simulink model "full_maneuver_platoon_new_strategy"  (R2019a)
settings: Solver=VariableStepAuto  StartTime=0.0  StopTime=70  FixedStep=0.1  MaxStep=0.05  RelTol=1e-3
libraries: simulink x97, dspsigops x7, powerlib_meascontrol x7, autolibshared x7
(part 1 of 7)
settings Model: Creator=fvall  LastModifiedBy=fvall

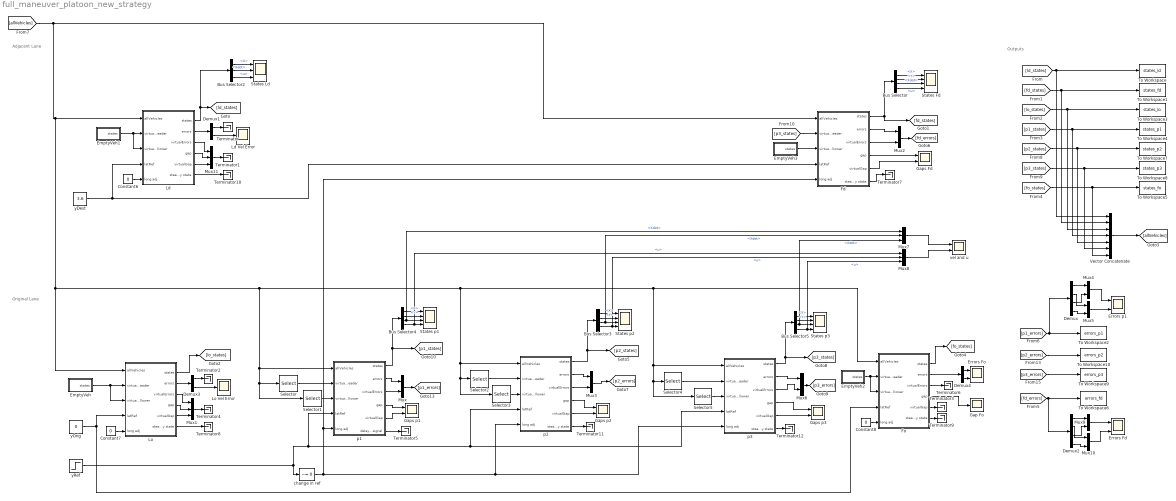
== system full_maneuver_platoon_new_strategy ==
  note: Adjacent Lane
  note: Outputs
  note: Original Lane
  Bus Selector{,3..5} (4 alike) : BusSelector  OutputSignals=X,Y,Xdot,u
  Bus Selector2 : BusSelector  OutputSignals=X,Xdot,u
  Constant6 : Constant  Value=0
  Constant7 : Constant  Value=0
  Constant8 : Constant  Value=0
  Demux : Demux
  Demux1 : Demux  Outputs=2
  Demux2 : Demux
  Demux3 : Demux  Outputs=2
  Demux4 : Demux  Outputs=2
  EmptyVeh : Subsystem
  EmptyVeh1 : Subsystem
  EmptyVeh2 : Subsystem
  EmptyVeh3 : Subsystem
  Errors Fd : Scope  NumInputPorts=2
  Errors Fo : Scope  NumInputPorts=2
  Errors p1 : Scope  NumInputPorts=2
  Fd : Subsystem  mask{m=2000, lf=2.5, lr=2.5, maxAcceleration=4, minAcceleration=-8, maxJerk=40, minJerk=-50, maxDelta=0.43633, maxDeltaDot=0.16406, freeFlowVel=29, A=[0 1 25 0;0 -0.92 0 -25.1;0 0 0 1;0 -0.05 0 -2.875], B=[0;12;0;15], C=[1 0 0 0;0 0 0 1], x0=40.2312, vx0=29, y0=3.6, h=0.63, d0=0.5004, minHeadwayError=-100, maxHeadwayError=3, velFilterGain=10, Kd=1.5652, Kp=2.2775, Ki=0.75, velKi=0.5, velKp=1.5, hFilterGain=0.5, vMin=18, maxComfAccel=2, minComfAccel=-2, maxComfJerk=10, minComfJerk=-10, hLc=2.1525, d0Lc=0.5004, Klat=[0.00909090909090922 0.00739381562390402 0.848484848484842 0.174418280834209], L=[12.1618468638973 6.0911647386398;-3.34743889176456 -72.8238882817198;1.29674659792577 4.97919690407453;0.0997536738638272 3.54315313610273]}
      mask prompts: m "autoblks_shared:autoblkVehBody3DofLat:blkPrm_m"; lf "autoblks_shared:autoblkVehBody3DofLat:blkPrm_a"; lr "autoblks_shared:autoblkVehBody3DofLat:blkPrm_b"; maxAcceleration "Max Acceleration"; minAcceleration "Min Acceleration"; maxJerk "Max Jerk"; minJerk "Min Jerk"; maxDelta "Max Delta"; maxDeltaDot "Max Delta Dot"; freeFlowVel "Free Flow Velocity"; x0 "autoblks_shared:autoblkVehBody3DofLat:blkPrm_X_o"; vx0 "autoblks_shared:autoblkVehBody3DofLat:blkPrm_xdot_o"; y0 "autoblks_shared:autoblkVehBody3DofLat:blkPrm_Y_o"; h "Time Headway"; d0 "Standstill Gap"; minHeadwayError "Min Headway Error"; maxHeadwayError "Max Headway Error"; velFilterGain "Velocity Filter Gain"; hFilterGain "Headway filter Gain"; vMin "Min velocity"; maxComfAccel "Max Comf Accel"; minComfAccel "Min Comf Accel"; maxComfJerk "Max Comf Jerk"; minComfJerk "Min Comf Jerk"; hLc "Time Headway LC"; d0Lc "Standstill Gap LC"; Klat "Lat Controller Gain"; L "Observer Gain"
      mask TypeOptions m: Vehicle Body 3DOF Single Track/m
      mask TypeOptions lf: Vehicle Body 3DOF Single Track/a
      mask TypeOptions lr: Vehicle Body 3DOF Single Track/b
      mask TypeOptions maxDelta: Lateral Control/Saturation/UpperLimit
      mask TypeOptions maxDeltaDot: Lateral Control/Rate Limiter/RisingSlewLimit
      mask TypeOptions A:
      | Lateral Control/Full State
      | Observer/Gain3/Gain
      mask TypeOptions B:
      | Lateral Control/Full State
      | Observer/Gain/Gain
      mask TypeOptions C:
      | Lateral Control/Full State
      | Observer/Gain1/Gain
      mask TypeOptions x0: Vehicle Body 3DOF Single Track/X_o
      mask TypeOptions vx0: Vehicle Body 3DOF Single Track/xdot_o
      mask TypeOptions y0: Vehicle Body 3DOF Single Track/Y_o
      mask TypeOptions h:
      | Regular Vehicle
      | Following/Compute Errors/h/Value
      mask TypeOptions d0:
      | Regular Vehicle
      | Following/Compute Errors/d0/Value
      mask TypeOptions Klat: Lateral Control/Gain1/Gain
      mask TypeOptions L:
      | Lateral Control/Full State
      | Observer/Gain2/Gain
      mask DialogControl DescGroupVar Prompt: 3DOF Vehicle with ACC
      mask DialogControl DescTextVar Prompt: Vehicle with ACC. The vehicle model is Simulink's 3DOF single track vehicle body. The controller is a PID with constant headway including headway error saturation and filtered leader velocity.
      mask DialogControl VehParams Prompt: Vehicle Parameters
      mask DialogControl m Prompt: Vehicle mass, m [kg]:
      mask DialogControl lf Prompt: Longitudinal distance from center of mass to front axle, a [m]:
      mask DialogControl lr Prompt: Longitudinal distance from center of mass to rear axle, b [m]:
      mask DialogControl latLinearModel Prompt: Lat Linear Model
      mask DialogControl InitStates Prompt: Initial State
      mask DialogControl x0 Prompt: Initial inertial frame longitudinal position, X_o [m]:
      mask DialogControl vx0 Prompt: Initial longitudinal velocity, xdot_o [m/s]:
      mask DialogControl y0 Prompt: Initial inertial frame lateral displacement, Y_o [m]:
      mask DialogControl Container3 Prompt: Veh Following Parameters
      mask DialogControl VirtualFollParams Prompt: Virtual Veh Following Parameters
      mask DialogControl LCParams Prompt: Lane Change Params
  Fo : Subsystem  mask{m=2000, lf=2.5, lr=2.5, maxAcceleration=4, minAcceleration=-8, maxJerk=40, minJerk=-50, maxDelta=0.43633, maxDeltaDot=0.16406, freeFlowVel=25, A=[0 1 25 0;0 -0.92 0 -25.1;0 0 0 1;0 -0.05 0 -2.875], B=[0;12;0;15], C=[1 0 0 0;0 0 0 1], x0=0, vx0=25, y0=0, h=0.63, d0=0.5004, minHeadwayError=-100, maxHeadwayError=3, velFilterGain=10, Kd=1.5652, Kp=2.2775, Ki=0.75, velKi=0.5, velKp=1.5, hFilterGain=0.5, vMin=18, maxComfAccel=2, minComfAccel=-2, maxComfJerk=10, minComfJerk=-10, hLc=1.9025, d0Lc=0.5004, Klat=[0.00909090909090922 0.00739381562390402 0.848484848484842 0.174418280834209], L=[12.1618468638973 6.0911647386398;-3.34743889176456 -72.8238882817198;1.29674659792577 4.97919690407453;0.0997536738638272 3.54315313610273]}
      mask prompts: m "autoblks_shared:autoblkVehBody3DofLat:blkPrm_m"; lf "autoblks_shared:autoblkVehBody3DofLat:blkPrm_a"; lr "autoblks_shared:autoblkVehBody3DofLat:blkPrm_b"; maxAcceleration "Max Acceleration"; minAcceleration "Min Acceleration"; maxJerk "Max Jerk"; minJerk "Min Jerk"; maxDelta "Max Delta"; maxDeltaDot "Max Delta Dot"; freeFlowVel "Free Flow Velocity"; x0 "autoblks_shared:autoblkVehBody3DofLat:blkPrm_X_o"; vx0 "autoblks_shared:autoblkVehBody3DofLat:blkPrm_xdot_o"; y0 "autoblks_shared:autoblkVehBody3DofLat:blkPrm_Y_o"; h "Time Headway"; d0 "Standstill Gap"; minHeadwayError "Min Headway Error"; maxHeadwayError "Max Headway Error"; velFilterGain "Velocity Filter Gain"; hFilterGain "Headway filter Gain"; vMin "Min velocity"; maxComfAccel "Max Comf Accel"; minComfAccel "Min Comf Accel"; maxComfJerk "Max Comf Jerk"; minComfJerk "Min Comf Jerk"; hLc "Time Headway LC"; d0Lc "Standstill Gap LC"; Klat "Lat Controller Gain"; L "Observer Gain"
      mask TypeOptions m: Vehicle Body 3DOF Single Track/m
      mask TypeOptions lf: Vehicle Body 3DOF Single Track/a
      mask TypeOptions lr: Vehicle Body 3DOF Single Track/b
      mask TypeOptions maxDelta: Lateral Control/Saturation/UpperLimit
      mask TypeOptions maxDeltaDot: Lateral Control/Rate Limiter/RisingSlewLimit
      mask TypeOptions A:
      | Lateral Control/Full State
      | Observer/Gain3/Gain
      mask TypeOptions B:
      | Lateral Control/Full State
      | Observer/Gain/Gain
      mask TypeOptions C:
      | Lateral Control/Full State
      | Observer/Gain1/Gain
      mask TypeOptions x0: Vehicle Body 3DOF Single Track/X_o
      mask TypeOptions vx0: Vehicle Body 3DOF Single Track/xdot_o
      mask TypeOptions y0: Vehicle Body 3DOF Single Track/Y_o
      mask TypeOptions h:
      | Regular Vehicle
      | Following/Compute Errors/h/Value
      mask TypeOptions d0:
      | Regular Vehicle
      | Following/Compute Errors/d0/Value
      mask TypeOptions vMin:
      | Longitudinal Adjustments
      | for Lane Change/Virtual Leader Following/vMin/Value
      mask TypeOptions Klat: Lateral Control/Gain1/Gain
      mask TypeOptions L:
      | Lateral Control/Full State
      | Observer/Gain2/Gain
      mask DialogControl DescGroupVar Prompt: 3DOF Vehicle with ACC
      mask DialogControl DescTextVar Prompt: Vehicle with ACC. The vehicle model is Simulink's 3DOF single track vehicle body. The controller is a PID with constant headway including headway error saturation and filtered leader velocity.
      mask DialogControl VehParams Prompt: Vehicle Parameters
      mask DialogControl m Prompt: Vehicle mass, m [kg]:
      mask DialogControl lf Prompt: Longitudinal distance from center of mass to front axle, a [m]:
      mask DialogControl lr Prompt: Longitudinal distance from center of mass to rear axle, b [m]:
      mask DialogControl latLinearModel Prompt: Lat Linear Model
      mask DialogControl InitStates Prompt: Initial State
      mask DialogControl x0 Prompt: Initial inertial frame longitudinal position, X_o [m]:
      mask DialogControl vx0 Prompt: Initial longitudinal velocity, xdot_o [m/s]:
      mask DialogControl y0 Prompt: Initial inertial frame lateral displacement, Y_o [m]:
      mask DialogControl Container3 Prompt: Veh Following Parameters
      mask DialogControl VirtualFollParams Prompt: Virtual Veh Following Parameters
      mask DialogControl LCParams Prompt: Lane Change Params
  Gap Fo : Scope
  Gaps Fd : Scope  NumInputPorts=2
  Gaps p1 : Scope  NumInputPorts=2
  Gaps p2 : Scope  NumInputPorts=2
  Gaps p3 : Scope  NumInputPorts=2
  Ld : Subsystem  mask{m=2000, lf=2.5, lr=2.5, maxAcceleration=4, minAcceleration=-8, maxJerk=40, minJerk=-50, maxDelta=0.43633, maxDeltaDot=0.16406, freeFlowVel=29, A=[0 1 25 0;0 -0.92 0 -25.1;0 0 0 1;0 -0.05 0 -2.875], B=[0;12;0;15], C=[1 0 0 0;0 0 0 1], x0=64.0016, vx0=29, y0=3.6, h=0.63, d0=0.5004, minHeadwayError=-100, maxHeadwayError=3, velFilterGain=10, Kd=1.5652, Kp=2.2775, Ki=0.75, velKi=0.5, velKp=1.5, hFilterGain=0.5, vMin=18, maxComfAccel=2, minComfAccel=-2, maxComfJerk=10, minComfJerk=-10, hLc=2.1525, d0Lc=0.5004, Klat=[0.00909090909090922 0.00739381562390402 0.848484848484842 0.174418280834209], L=[12.1618468638973 6.0911647386398;-3.34743889176456 -72.8238882817198;1.29674659792577 4.97919690407453;0.0997536738638272 3.54315313610273]}
      mask prompts: m "autoblks_shared:autoblkVehBody3DofLat:blkPrm_m"; lf "autoblks_shared:autoblkVehBody3DofLat:blkPrm_a"; lr "autoblks_shared:autoblkVehBody3DofLat:blkPrm_b"; maxAcceleration "Max Acceleration"; minAcceleration "Min Acceleration"; maxJerk "Max Jerk"; minJerk "Min Jerk"; maxDelta "Max Delta"; maxDeltaDot "Max Delta Dot"; freeFlowVel "Free Flow Velocity"; x0 "autoblks_shared:autoblkVehBody3DofLat:blkPrm_X_o"; vx0 "autoblks_shared:autoblkVehBody3DofLat:blkPrm_xdot_o"; y0 "autoblks_shared:autoblkVehBody3DofLat:blkPrm_Y_o"; h "Time Headway"; d0 "Standstill Gap"; minHeadwayError "Min Headway Error"; maxHeadwayError "Max Headway Error"; velFilterGain "Velocity Filter Gain"; hFilterGain "Headway filter Gain"; vMin "Min velocity"; maxComfAccel "Max Comf Accel"; minComfAccel "Min Comf Accel"; maxComfJerk "Max Comf Jerk"; minComfJerk "Min Comf Jerk"; hLc "Time Headway LC"; d0Lc "Standstill Gap LC"; Klat "Lat Controller Gain"; L "Observer Gain"
      mask TypeOptions m: Vehicle Body 3DOF Single Track/m
      mask TypeOptions lf: Vehicle Body 3DOF Single Track/a
      mask TypeOptions lr: Vehicle Body 3DOF Single Track/b
      mask TypeOptions maxDelta: Lateral Control/Saturation/UpperLimit
      mask TypeOptions maxDeltaDot: Lateral Control/Rate Limiter/RisingSlewLimit
      mask TypeOptions A:
      | Lateral Control/Full State
      | Observer/Gain3/Gain
      mask TypeOptions B:
      | Lateral Control/Full State
      | Observer/Gain/Gain
      mask TypeOptions C:
      | Lateral Control/Full State
      | Observer/Gain1/Gain
      mask TypeOptions x0: Vehicle Body 3DOF Single Track/X_o
      mask TypeOptions vx0: Vehicle Body 3DOF Single Track/xdot_o
      mask TypeOptions y0: Vehicle Body 3DOF Single Track/Y_o
      mask TypeOptions h:
      | Regular Vehicle
      | Following/Compute Errors/h/Value
      mask TypeOptions d0:
      | Regular Vehicle
      | Following/Compute Errors/d0/Value
      mask TypeOptions Klat: Lateral Control/Gain1/Gain
      mask TypeOptions L:
      | Lateral Control/Full State
      | Observer/Gain2/Gain
      mask DialogControl DescGroupVar Prompt: 3DOF Vehicle with ACC
      mask DialogControl DescTextVar Prompt: Vehicle with ACC. The vehicle model is Simulink's 3DOF single track vehicle body. The controller is a PID with constant headway including headway error saturation and filtered leader velocity.
      mask DialogControl VehParams Prompt: Vehicle Parameters
      mask DialogControl m Prompt: Vehicle mass, m [kg]:
      mask DialogControl lf Prompt: Longitudinal distance from center of mass to front axle, a [m]:
      mask DialogControl lr Prompt: Longitudinal distance from center of mass to rear axle, b [m]:
      mask DialogControl latLinearModel Prompt: Lat Linear Model
      mask DialogControl InitStates Prompt: Initial State
      mask DialogControl x0 Prompt: Initial inertial frame longitudinal position, X_o [m]:
      mask DialogControl vx0 Prompt: Initial longitudinal velocity, xdot_o [m/s]:
      mask DialogControl y0 Prompt: Initial inertial frame lateral displacement, Y_o [m]:
      mask DialogControl Container3 Prompt: Veh Following Parameters
      mask DialogControl VirtualFollParams Prompt: Virtual Veh Following Parameters
      mask DialogControl LCParams Prompt: Lane Change Params
  Ld Vel Error : Scope
  Lo : Subsystem  mask{m=2000, lf=2.5, lr=2.5, maxAcceleration=4, minAcceleration=-8, maxJerk=40, minJerk=-50, maxDelta=0.43633, maxDeltaDot=0.16406, freeFlowVel=25, A=[0 1 25 0;0 -0.92 0 -25.1;0 0 0 1;0 -0.05 0 -2.875], B=[0;12;0;15], C=[1 0 0 0;0 0 0 1], x0=85.0016, vx0=25, y0=0, h=0.63, d0=0.5004, minHeadwayError=-100, maxHeadwayError=3, velFilterGain=10, Kd=1.5652, Kp=2.2775, Ki=0.75, velKi=0.5, velKp=1.5, hFilterGain=0.5, vMin=18, maxComfAccel=2, minComfAccel=-2, maxComfJerk=10, minComfJerk=-10, hLc=1.9025, d0Lc=0.5004, Klat=[0.00909090909090922 0.00739381562390402 0.848484848484842 0.174418280834209], L=[12.1618468638973 6.0911647386398;-3.34743889176456 -72.8238882817198;1.29674659792577 4.97919690407453;0.0997536738638272 3.54315313610273]}
      mask prompts: m "autoblks_shared:autoblkVehBody3DofLat:blkPrm_m"; lf "autoblks_shared:autoblkVehBody3DofLat:blkPrm_a"; lr "autoblks_shared:autoblkVehBody3DofLat:blkPrm_b"; maxAcceleration "Max Acceleration"; minAcceleration "Min Acceleration"; maxJerk "Max Jerk"; minJerk "Min Jerk"; maxDelta "Max Delta"; maxDeltaDot "Max Delta Dot"; freeFlowVel "Free Flow Velocity"; x0 "autoblks_shared:autoblkVehBody3DofLat:blkPrm_X_o"; vx0 "autoblks_shared:autoblkVehBody3DofLat:blkPrm_xdot_o"; y0 "autoblks_shared:autoblkVehBody3DofLat:blkPrm_Y_o"; h "Time Headway"; d0 "Standstill Gap"; minHeadwayError "Min Headway Error"; maxHeadwayError "Max Headway Error"; velFilterGain "Velocity Filter Gain"; hFilterGain "Headway filter Gain"; vMin "Min velocity"; maxComfAccel "Max Comf Accel"; minComfAccel "Min Comf Accel"; maxComfJerk "Max Comf Jerk"; minComfJerk "Min Comf Jerk"; hLc "Time Headway LC"; d0Lc "Standstill Gap LC"; Klat "Lat Controller Gain"; L "Observer Gain"
      mask TypeOptions m: Vehicle Body 3DOF Single Track/m
      mask TypeOptions lf: Vehicle Body 3DOF Single Track/a
      mask TypeOptions lr: Vehicle Body 3DOF Single Track/b
      mask TypeOptions maxDelta: Lateral Control/Saturation/UpperLimit
      mask TypeOptions maxDeltaDot: Lateral Control/Rate Limiter/RisingSlewLimit
      mask TypeOptions A:
      | Lateral Control/Full State
      | Observer/Gain3/Gain
      mask TypeOptions B:
      | Lateral Control/Full State
      | Observer/Gain/Gain
      mask TypeOptions C:
      | Lateral Control/Full State
      | Observer/Gain1/Gain
      mask TypeOptions x0: Vehicle Body 3DOF Single Track/X_o
      mask TypeOptions vx0: Vehicle Body 3DOF Single Track/xdot_o
      mask TypeOptions y0: Vehicle Body 3DOF Single Track/Y_o
      mask TypeOptions h:
      | Regular Vehicle
      | Following/Compute Errors/h/Value
      mask TypeOptions d0:
      | Regular Vehicle
      | Following/Compute Errors/d0/Value
      mask TypeOptions Klat: Lateral Control/Gain1/Gain
      mask TypeOptions L:
      | Lateral Control/Full State
      | Observer/Gain2/Gain
      mask DialogControl DescGroupVar Prompt: 3DOF Vehicle with ACC
      mask DialogControl DescTextVar Prompt: Vehicle with ACC. The vehicle model is Simulink's 3DOF single track vehicle body. The controller is a PID with constant headway including headway error saturation and filtered leader velocity.
      mask DialogControl VehParams Prompt: Vehicle Parameters
      mask DialogControl m Prompt: Vehicle mass, m [kg]:
      mask DialogControl lf Prompt: Longitudinal distance from center of mass to front axle, a [m]:
      mask DialogControl lr Prompt: Longitudinal distance from center of mass to rear axle, b [m]:
      mask DialogControl latLinearModel Prompt: Lat Linear Model
      mask DialogControl InitStates Prompt: Initial State
      mask DialogControl x0 Prompt: Initial inertial frame longitudinal position, X_o [m]:
      mask DialogControl vx0 Prompt: Initial longitudinal velocity, xdot_o [m/s]:
      mask DialogControl y0 Prompt: Initial inertial frame lateral displacement, Y_o [m]:
      mask DialogControl Container3 Prompt: Veh Following Parameters
      mask DialogControl VirtualFollParams Prompt: Virtual Veh Following Parameters
      mask DialogControl LCParams Prompt: Lane Change Params
  Lo Vel Error : Scope
  Mux{,2..6,9..10} (8 alike) : Mux  Inputs=2
  Mux{1,7..8,11} (4 alike) : Mux  Inputs=3
  Selector : Selector  InputPortWidth=7  IndexOptions=Index vector (dialog)  Indices=[1]  OutputSizes=1
  Selector1 : Selector  InputPortWidth=7  IndexOptions=Index vector (dialog)  Indices=[2]  OutputSizes=1
  Selector2 : Selector  InputPortWidth=7  IndexOptions=Index vector (dialog)  Indices=[4]  OutputSizes=1
  Selector3 : Selector  InputPortWidth=7  IndexOptions=Index vector (dialog)  Indices=[2]  OutputSizes=1
  Selector4 : Selector  InputPortWidth=7  IndexOptions=Index vector (dialog)  Indices=[5]  OutputSizes=1
  Selector5 : Selector  InputPortWidth=7  IndexOptions=Index vector (dialog)  Indices=[2]  OutputSizes=1
  States Fd : Scope  NumInputPorts=4
  States Ld : Scope  NumInputPorts=3
  States p1 : Scope  NumInputPorts=4
  States p2 : Scope  NumInputPorts=4
  States p3 : Scope  NumInputPorts=4
  Terminator{,1..12} (13 alike) : Terminator
  To Workspace : ToWorkspace  VariableName=states_ld  SaveFormat=Timeseries  SampleTime=-1
  To Workspace1 : ToWorkspace  VariableName=states_fd  SaveFormat=Timeseries  SampleTime=-1
  To Workspace10 : ToWorkspace  VariableName=errors_p2  SampleTime=-1
  To Workspace2 : ToWorkspace  VariableName=errors_p1  SampleTime=-1
  To Workspace3 : ToWorkspace  VariableName=states_lo  SaveFormat=Timeseries  SampleTime=-1
  To Workspace4 : ToWorkspace  VariableName=states_p1  SaveFormat=Timeseries  SampleTime=-1
  To Workspace5 : ToWorkspace  VariableName=states_fo  SaveFormat=Timeseries  SampleTime=-1
  To Workspace6 : ToWorkspace  VariableName=errors_fd  SampleTime=-1
  To Workspace7 : ToWorkspace  VariableName=states_p2  SaveFormat=Timeseries  SampleTime=-1
  To Workspace8 : ToWorkspace  VariableName=states_p3  SaveFormat=Timeseries  SampleTime=-1
  To Workspace9 : ToWorkspace  VariableName=errors_p3  SampleTime=-1
  Vector Concatenate : Concatenate  NumInputs=7
  change in ref : simulink/Logic and Bit Operations/Compare To Constant  relop=~=  const=0  OutDataTypeStr=boolean
  p1 : Subsystem  mask{m=2000, lf=2.5, lr=2.5, maxAcceleration=4, minAcceleration=-8, maxJerk=40, minJerk=-50, maxDelta=0.43633, maxDeltaDot=0.16406, freeFlowVel=25, A=[0 1 25 0;0 -0.92 0 -25.1;0 0 0 1;0 -0.05 0 -2.875], B=[0;12;0;15], C=[1 0 0 0;0 0 0 1], x0=63.7512, vx0=25, y0=0, h=0.63, d0=0.5004, minHeadwayError=-100, maxHeadwayError=3, velFilterGain=10, Kd=1.5652, Kp=2.2775, Ki=0.75, velKi=0.5, velKp=1.5, hFilterGain=0.5, vMin=18, maxComfAccel=2, minComfAccel=-2, maxComfJerk=10, minComfJerk=-10, hLc=1.9025, d0Lc=0.5004, Klat=[0.00909090909090922 0.00739381562390402 0.848484848484842 0.174418280834209], L=[12.1618468638973 6.0911647386398;-3.34743889176456 -72.8238882817198;1.29674659792577 4.97919690407453;0.0997536738638272 3.54315313610273]}
      mask prompts: m "autoblks_shared:autoblkVehBody3DofLat:blkPrm_m"; lf "autoblks_shared:autoblkVehBody3DofLat:blkPrm_a"; lr "autoblks_shared:autoblkVehBody3DofLat:blkPrm_b"; maxAcceleration "Max Acceleration"; minAcceleration "Min Acceleration"; maxJerk "Max Jerk"; minJerk "Min Jerk"; maxDelta "Max Delta"; maxDeltaDot "Max Delta Dot"; freeFlowVel "Free Flow Velocity"; x0 "autoblks_shared:autoblkVehBody3DofLat:blkPrm_X_o"; vx0 "autoblks_shared:autoblkVehBody3DofLat:blkPrm_xdot_o"; y0 "autoblks_shared:autoblkVehBody3DofLat:blkPrm_Y_o"; h "Time Headway"; d0 "Standstill Gap"; minHeadwayError "Min Headway Error"; maxHeadwayError "Max Headway Error"; velFilterGain "Velocity Filter Gain"; hFilterGain "Headway filter Gain"; vMin "Min velocity"; maxComfAccel "Max Comf Accel"; minComfAccel "Min Comf Accel"; maxComfJerk "Max Comf Jerk"; minComfJerk "Min Comf Jerk"; hLc "Time Headway LC"; d0Lc "Standstill Gap LC"; Klat "Lat Controller Gain"; L "Observer Gain"
      mask TypeOptions m: Vehicle Body 3DOF Single Track/m
      mask TypeOptions lf: Vehicle Body 3DOF Single Track/a
      mask TypeOptions lr: Vehicle Body 3DOF Single Track/b
      mask TypeOptions maxDelta: Lateral Control/Saturation/UpperLimit
      mask TypeOptions maxDeltaDot: Lateral Control/Rate Limiter/RisingSlewLimit
      mask TypeOptions A:
      | Lateral Control/Full State
      | Observer/Gain3/Gain
      mask TypeOptions B:
      | Lateral Control/Full State
      | Observer/Gain/Gain
      mask TypeOptions C:
      | Lateral Control/Full State
      | Observer/Gain1/Gain
      mask TypeOptions x0: Vehicle Body 3DOF Single Track/X_o
      mask TypeOptions vx0: Vehicle Body 3DOF Single Track/xdot_o
      mask TypeOptions y0: Vehicle Body 3DOF Single Track/Y_o
      mask TypeOptions h:
      | Regular Vehicle
      | Following/Compute Errors/h/Value
      mask TypeOptions d0:
      | Regular Vehicle
      | Following/Compute Errors/d0/Value
      mask TypeOptions Klat: Lateral Control/Gain1/Gain
      mask TypeOptions L:
      | Lateral Control/Full State
      | Observer/Gain2/Gain
      mask DialogControl DescGroupVar Prompt: 3DOF Vehicle with ACC
      mask DialogControl DescTextVar Prompt: Vehicle with ACC. The vehicle model is Simulink's 3DOF single track vehicle body. The controller is a PID with constant headway including headway error saturation and filtered leader velocity.
      mask DialogControl VehParams Prompt: Vehicle Parameters
      mask DialogControl m Prompt: Vehicle mass, m [kg]:
      mask DialogControl lf Prompt: Longitudinal distance from center of mass to front axle, a [m]:
      mask DialogControl lr Prompt: Longitudinal distance from center of mass to rear axle, b [m]:
      mask DialogControl latLinearModel Prompt: Lat Linear Model
      mask DialogControl InitStates Prompt: Initial State
      mask DialogControl x0 Prompt: Initial inertial frame longitudinal position, X_o [m]:
      mask DialogControl vx0 Prompt: Initial longitudinal velocity, xdot_o [m/s]:
      mask DialogControl y0 Prompt: Initial inertial frame lateral displacement, Y_o [m]:
      mask DialogControl Container3 Prompt: Veh Following Parameters
      mask DialogControl VirtualFollParams Prompt: Virtual Veh Following Parameters
      mask DialogControl LCParams Prompt: Lane Change Params
  p2 : Subsystem  mask{m=2000, lf=2.5, lr=2.5, maxAcceleration=4, minAcceleration=-8, maxJerk=40, minJerk=-50, maxDelta=0.43633, maxDeltaDot=0.16406, freeFlowVel=25, A=[0 1 25 0;0 -0.92 0 -25.1;0 0 0 1;0 -0.05 0 -2.875], B=[0;12;0;15], C=[1 0 0 0;0 0 0 1], x0=42.5008, vx0=25, y0=0, h=0.63, d0=0.5004, minHeadwayError=-100, maxHeadwayError=3, velFilterGain=10, Kd=1.5652, Kp=2.2775, Ki=0.75, velKi=0.5, velKp=1.5, hFilterGain=0.5, vMin=18, maxComfAccel=2, minComfAccel=-2, maxComfJerk=10, minComfJerk=-10, hLc=1.9025, d0Lc=0.5004, Klat=[0.00909090909090922 0.00739381562390402 0.848484848484842 0.174418280834209], L=[12.1618468638973 6.0911647386398;-3.34743889176456 -72.8238882817198;1.29674659792577 4.97919690407453;0.0997536738638272 3.54315313610273]}
      mask prompts: m "autoblks_shared:autoblkVehBody3DofLat:blkPrm_m"; lf "autoblks_shared:autoblkVehBody3DofLat:blkPrm_a"; lr "autoblks_shared:autoblkVehBody3DofLat:blkPrm_b"; maxAcceleration "Max Acceleration"; minAcceleration "Min Acceleration"; maxJerk "Max Jerk"; minJerk "Min Jerk"; maxDelta "Max Delta"; maxDeltaDot "Max Delta Dot"; freeFlowVel "Free Flow Velocity"; x0 "autoblks_shared:autoblkVehBody3DofLat:blkPrm_X_o"; vx0 "autoblks_shared:autoblkVehBody3DofLat:blkPrm_xdot_o"; y0 "autoblks_shared:autoblkVehBody3DofLat:blkPrm_Y_o"; h "Time Headway"; d0 "Standstill Gap"; minHeadwayError "Min Headway Error"; maxHeadwayError "Max Headway Error"; velFilterGain "Velocity Filter Gain"; hFilterGain "Headway filter Gain"; vMin "Min velocity"; maxComfAccel "Max Comf Accel"; minComfAccel "Min Comf Accel"; maxComfJerk "Max Comf Jerk"; minComfJerk "Min Comf Jerk"; hLc "Time Headway LC"; d0Lc "Standstill Gap LC"; Klat "Lat Controller Gain"; L "Observer Gain"
      mask TypeOptions m: Vehicle Body 3DOF Single Track/m
      mask TypeOptions lf: Vehicle Body 3DOF Single Track/a
      mask TypeOptions lr: Vehicle Body 3DOF Single Track/b
      mask TypeOptions maxDelta: Lateral Control/Saturation/UpperLimit
      mask TypeOptions maxDeltaDot: Lateral Control/Rate Limiter/RisingSlewLimit
      mask TypeOptions A:
      | Lateral Control/Full State
      | Observer/Gain3/Gain
      mask TypeOptions B:
      | Lateral Control/Full State
      | Observer/Gain/Gain
      mask TypeOptions C:
      | Lateral Control/Full State
      | Observer/Gain1/Gain
      mask TypeOptions x0: Vehicle Body 3DOF Single Track/X_o
      mask TypeOptions vx0: Vehicle Body 3DOF Single Track/xdot_o
      mask TypeOptions y0: Vehicle Body 3DOF Single Track/Y_o
      mask TypeOptions h:
      | Regular Vehicle
      | Following/Compute Errors/h/Value
      mask TypeOptions d0:
      | Regular Vehicle
      | Following/Compute Errors/d0/Value
      mask TypeOptions Klat: Lateral Control/Gain1/Gain
      mask TypeOptions L:
      | Lateral Control/Full State
      | Observer/Gain2/Gain
      mask DialogControl DescGroupVar Prompt: 3DOF Vehicle with ACC
      mask DialogControl DescTextVar Prompt: Vehicle with ACC. The vehicle model is Simulink's 3DOF single track vehicle body. The controller is a PID with constant headway including headway error saturation and filtered leader velocity.
      mask DialogControl VehParams Prompt: Vehicle Parameters
      mask DialogControl m Prompt: Vehicle mass, m [kg]:
      mask DialogControl lf Prompt: Longitudinal distance from center of mass to front axle, a [m]:
      mask DialogControl lr Prompt: Longitudinal distance from center of mass to rear axle, b [m]:
      mask DialogControl latLinearModel Prompt: Lat Linear Model
      mask DialogControl InitStates Prompt: Initial State
      mask DialogControl x0 Prompt: Initial inertial frame longitudinal position, X_o [m]:
      mask DialogControl vx0 Prompt: Initial longitudinal velocity, xdot_o [m/s]:
      mask DialogControl y0 Prompt: Initial inertial frame lateral displacement, Y_o [m]:
      mask DialogControl Container3 Prompt: Veh Following Parameters
      mask DialogControl VirtualFollParams Prompt: Virtual Veh Following Parameters
      mask DialogControl LCParams Prompt: Lane Change Params
  p3 : Subsystem  mask{m=2000, lf=2.5, lr=2.5, maxAcceleration=4, minAcceleration=-8, maxJerk=40, minJerk=-50, maxDelta=0.43633, maxDeltaDot=0.16406, freeFlowVel=25, A=[0 1 25 0;0 -0.92 0 -25.1;0 0 0 1;0 -0.05 0 -2.875], B=[0;12;0;15], C=[1 0 0 0;0 0 0 1], x0=21.2504, vx0=25, y0=0, h=0.63, d0=0.5004, minHeadwayError=-100, maxHeadwayError=3, velFilterGain=10, Kd=1.5652, Kp=2.2775, Ki=0.75, velKi=0.5, velKp=1.5, hFilterGain=0.5, vMin=18, maxComfAccel=2, minComfAccel=-2, maxComfJerk=10, minComfJerk=-10, hLc=1.9025, d0Lc=0.5004, Klat=[0.00909090909090922 0.00739381562390402 0.848484848484842 0.174418280834209], L=[12.1618468638973 6.0911647386398;-3.34743889176456 -72.8238882817198;1.29674659792577 4.97919690407453;0.0997536738638272 3.54315313610273]}
      mask prompts: m "autoblks_shared:autoblkVehBody3DofLat:blkPrm_m"; lf "autoblks_shared:autoblkVehBody3DofLat:blkPrm_a"; lr "autoblks_shared:autoblkVehBody3DofLat:blkPrm_b"; maxAcceleration "Max Acceleration"; minAcceleration "Min Acceleration"; maxJerk "Max Jerk"; minJerk "Min Jerk"; maxDelta "Max Delta"; maxDeltaDot "Max Delta Dot"; freeFlowVel "Free Flow Velocity"; x0 "autoblks_shared:autoblkVehBody3DofLat:blkPrm_X_o"; vx0 "autoblks_shared:autoblkVehBody3DofLat:blkPrm_xdot_o"; y0 "autoblks_shared:autoblkVehBody3DofLat:blkPrm_Y_o"; h "Time Headway"; d0 "Standstill Gap"; minHeadwayError "Min Headway Error"; maxHeadwayError "Max Headway Error"; velFilterGain "Velocity Filter Gain"; hFilterGain "Headway filter Gain"; vMin "Min velocity"; maxComfAccel "Max Comf Accel"; minComfAccel "Min Comf Accel"; maxComfJerk "Max Comf Jerk"; minComfJerk "Min Comf Jerk"; hLc "Time Headway LC"; d0Lc "Standstill Gap LC"; Klat "Lat Controller Gain"; L "Observer Gain"
      mask TypeOptions m: Vehicle Body 3DOF Single Track/m
      mask TypeOptions lf: Vehicle Body 3DOF Single Track/a
      mask TypeOptions lr: Vehicle Body 3DOF Single Track/b
      mask TypeOptions maxDelta: Lateral Control/Saturation/UpperLimit
      mask TypeOptions maxDeltaDot: Lateral Control/Rate Limiter/RisingSlewLimit
      mask TypeOptions A:
      | Lateral Control/Full State
      | Observer/Gain3/Gain
      mask TypeOptions B:
      | Lateral Control/Full State
      | Observer/Gain/Gain
      mask TypeOptions C:
      | Lateral Control/Full State
      | Observer/Gain1/Gain
      mask TypeOptions x0: Vehicle Body 3DOF Single Track/X_o
      mask TypeOptions vx0: Vehicle Body 3DOF Single Track/xdot_o
      mask TypeOptions y0: Vehicle Body 3DOF Single Track/Y_o
      mask TypeOptions h:
      | Regular Vehicle
      | Following/Compute Errors/h/Value
      mask TypeOptions d0:
      | Regular Vehicle
      | Following/Compute Errors/d0/Value
      mask TypeOptions Klat: Lateral Control/Gain1/Gain
      mask TypeOptions L:
      | Lateral Control/Full State
      | Observer/Gain2/Gain
      mask DialogControl DescGroupVar Prompt: 3DOF Vehicle with ACC
      mask DialogControl DescTextVar Prompt: Vehicle with ACC. The vehicle model is Simulink's 3DOF single track vehicle body. The controller is a PID with constant headway including headway error saturation and filtered leader velocity.
      mask DialogControl VehParams Prompt: Vehicle Parameters
      mask DialogControl m Prompt: Vehicle mass, m [kg]:
      mask DialogControl lf Prompt: Longitudinal distance from center of mass to front axle, a [m]:
      mask DialogControl lr Prompt: Longitudinal distance from center of mass to rear axle, b [m]:
      mask DialogControl latLinearModel Prompt: Lat Linear Model
      mask DialogControl InitStates Prompt: Initial State
      mask DialogControl x0 Prompt: Initial inertial frame longitudinal position, X_o [m]:
      mask DialogControl vx0 Prompt: Initial longitudinal velocity, xdot_o [m/s]:
      mask DialogControl y0 Prompt: Initial inertial frame lateral displacement, Y_o [m]:
      mask DialogControl Container3 Prompt: Veh Following Parameters
      mask DialogControl VirtualFollParams Prompt: Virtual Veh Following Parameters
      mask DialogControl LCParams Prompt: Lane Change Params
  vel and u : Scope  NumInputPorts=2
  yDest : Constant  Value=3.6
  yOrig : Constant  Value=0
  yRef : Step  Time=5  After=3.6  SampleTime=0
  wires:
  Lo/2(errors) -> Demux3/1
  Fo/3(virtualErrors) -> Terminator6/1
  Lo/5(virtualGap) -> Mux1/3
  [p1_errors] -> To Workspace2/1, Demux/1
  Ld/3(virtualErrors) -> Mux11/1
  Lo/6(steady state) -> Terminator8/1
  Demux3/1 -> Terminator2/1
  Mux5/1 -> Errors p1/2
  Demux4/2 -> Errors Fo/2
  p1/3(virtualErrors) -> Mux/2
  Demux3/2 -> Lo Vel Error/1
  Bus Selector4/4 -> Mux8/1, States p1/4  "<u>"
  Lo/3(virtualErrors) -> Mux1/1
  p1/5(virtualGap) -> Gaps p1/2
  Mux1/1 -> Terminator4/1
  Demux2/2 -> Mux10/1
  Lo/4(gap) -> Mux1/2
  Demux1/1 -> Terminator/1
  Mux/1 -> [p1_errors]
  Ld/5(virtualGap) -> Mux11/3
  Demux/3 -> Mux4/2
  Fo/6(steady state) -> Terminator9/1
  Demux/1 -> Mux4/1
  [fo_states] -> To Workspace5/1, Vector Concatenate/7
  Ld/6(steady state) -> Terminator10/1
  Demux2/1 -> Mux9/1
  Demux/4 -> Mux5/2
  [ld_states] -> Vector Concatenate/1, To Workspace/1
  [p1_states] -> To Workspace4/1, Vector Concatenate/4
  [fd_errors] -> Demux2/1, To Workspace6/1
  Demux2/4 -> Mux10/2
  change in ref/1 -> p3/5(long adj), p2/5(long adj), Fd/5(long adj), p1/5(long adj)
  Demux2/3 -> Mux9/2
  Fd/3(virtualErrors) -> Mux2/2
  Demux/2 -> Mux5/1
  Mux9/1 -> Errors Fd/1
  Ld/2(errors) -> Demux1/1
  Demux4/1 -> Errors Fo/1
  Mux10/1 -> Errors Fd/2
  p1/1(states) -> Bus Selector4/1, [p1_states]
  Constant7/1 -> Lo/5(long adj)
  Fd/2(errors) -> Mux2/1
  Fo/5(virtualGap) -> Terminator3/1
  Fo/4(gap) -> Gap Fo/1
  Constant8/1 -> Fo/5(long adj)
  Fo/1(states) -> [fo_states]
  [lo_states] -> Vector Concatenate/3, To Workspace3/1
  Fo/2(errors) -> Demux4/1
  Constant6/1 -> Ld/5(long adj)
  Mux2/1 -> [fd_errors]
  Ld/4(gap) -> Mux11/2
  Bus Selector/3 -> States Fd/3  "<Xdot>"
  Lo/1(states) -> [lo_states]
  p1/4(gap) -> Gaps p1/1
  [fd_states] -> Vector Concatenate/2, To Workspace1/1
  Mux4/1 -> Errors p1/1
  Bus Selector/4 -> States Fd/4  "<u>"
  Fd/5(virtualGap) -> Gaps Fd/2
  [p3_states] -> Fd/2(virtualLeader)
  Bus Selector2/2 -> States Ld/2  "<Xdot>"
  Bus Selector/1 -> States Fd/1  "<X>"
  Bus Selector2/1 -> States Ld/1  "<X>"
  Bus Selector4/1 -> States p1/1  "<X>"
  Demux1/2 -> Ld Vel Error/1
  Mux11/1 -> Terminator1/1
  Fd/4(gap) -> Gaps Fd/1
  Fd/1(states) -> [fd_states], Bus Selector/1
  Selector/1 -> p1/2(virtualLeader)
  Fd/6(steady state) -> Terminator7/1
  p1/2(errors) -> Mux/1
  Ld/1(states) -> Bus Selector2/1, [ld_states]
  Bus Selector2/3 -> States Ld/3  "<u>"
  Bus Selector4/3 -> Mux7/1, States p1/3  "<Xdot>"
  Bus Selector4/2 -> States p1/2  "<Y>"
  yRef/1 -> p1/4(latRef), p3/4(latRef), p2/4(latRef), change in ref/1
  yDest/1 -> Fd/4(latRef), Ld/4(latRef)
  yOrig/1 -> Fo/4(latRef), Lo/4(latRef)
  Bus Selector/2 -> States Fd/2  "<Y>"
  [allVehicles] -> Fd/1(allVehicles), Lo/1(allVehicles), p1/1(allVehicles), Selector/1, Selector1/1, Fo/1(allVehicles), p3/1(allVehicles), Selector5/1, Selector4/1, Selector3/1, Selector2/1, p2/1(allVehicles), Ld/1(allVehicles)
  Vector Concatenate/1 -> [allVehicles]
  EmptyVeh/1(states) -> Lo/3(virtualFollower), Lo/2(virtualLeader)
  EmptyVeh1/1(states) -> Ld/3(virtualFollower), Ld/2(virtualLeader)
  Selector1/1 -> p1/3(virtualFollower)
  EmptyVeh3/1(states) -> Fd/3(virtualFollower)
  EmptyVeh2/1(states) -> Fo/3(virtualFollower), Fo/2(virtualLeader)
  p2/4(gap) -> Gaps p2/1
  p2/3(virtualErrors) -> Mux3/2
  Bus Selector3/4 -> Mux8/2, States p2/4  "<u>"
  p2/5(virtualGap) -> Gaps p2/2
  p2/1(states) -> Bus Selector3/1, [p2_states]
  p2/2(errors) -> Mux3/1
  Mux3/1 -> [p2_errors]
  Bus Selector3/1 -> States p2/1  "<X>"
  Bus Selector3/3 -> Mux7/2, States p2/3  "<Xdot>"
  Bus Selector3/2 -> States p2/2  "<Y>"
  Bus Selector5/3 -> Mux7/3, States p3/3  "<Xdot>"
  Mux6/1 -> [p3_errors]
  Bus Selector5/2 -> States p3/2  "<Y>"
  p3/2(errors) -> Mux6/1
  p3/6(steady state) -> Terminator12/1
  p3/3(virtualErrors) -> Mux6/2
  p3/1(states) -> Bus Selector5/1, [p3_states]
  p3/5(virtualGap) -> Gaps p3/2
  p3/4(gap) -> Gaps p3/1
  Bus Selector5/4 -> Mux8/3, States p3/4  "<u>"
  Bus Selector5/1 -> States p3/1  "<X>"
  Selector3/1 -> p2/3(virtualFollower)
  Selector2/1 -> p2/2(virtualLeader)
  [p2_states] -> Vector Concatenate/5, To Workspace7/1
  [p3_states] -> Vector Concatenate/6, To Workspace8/1
  Selector4/1 -> p3/2(virtualLeader)
  Selector5/1 -> p3/3(virtualFollower)
  [p3_errors] -> To Workspace9/1
  [p2_errors] -> To Workspace10/1
  Mux7/1 -> vel and u/1
  Mux8/1 -> vel and u/2
  p1/6(delayedLCsignal) -> Terminator5/1
  p2/6(steady state) -> Terminator11/1

== system full_maneuver_platoon_new_strategy/EmptyVeh ==
  Bus Creator1 : BusCreator  Inputs=4  OutDataTypeStr=Bus: vehStatesBus
  Constant{,1..3} (4 alike) : Constant  Value=0
  states : Outport
  wires:
  Constant3/1 -> Bus Creator1/4  "u"
  Bus Creator1/1 -> states/1
  Constant1/1 -> Bus Creator1/1  "X"
  Constant2/1 -> Bus Creator1/3  "Xdot"
  Constant/1 -> Bus Creator1/2  "Y"

== system full_maneuver_platoon_new_strategy/EmptyVeh1 ==
  Bus Creator1 : BusCreator  Inputs=4  OutDataTypeStr=Bus: vehStatesBus
  Constant{,1..3} (4 alike) : Constant  Value=0
  states : Outport
  wires:
  Constant3/1 -> Bus Creator1/4  "u"
  Bus Creator1/1 -> states/1
  Constant1/1 -> Bus Creator1/1  "X"
  Constant2/1 -> Bus Creator1/3  "Xdot"
  Constant/1 -> Bus Creator1/2  "Y"

== system full_maneuver_platoon_new_strategy/EmptyVeh2 ==
  Bus Creator1 : BusCreator  Inputs=4  OutDataTypeStr=Bus: vehStatesBus
  Constant{,1..3} (4 alike) : Constant  Value=0
  states : Outport
  wires:
  Constant3/1 -> Bus Creator1/4  "u"
  Bus Creator1/1 -> states/1
  Constant1/1 -> Bus Creator1/1  "X"
  Constant2/1 -> Bus Creator1/3  "Xdot"
  Constant/1 -> Bus Creator1/2  "Y"

== system full_maneuver_platoon_new_strategy/EmptyVeh3 ==
  Bus Creator1 : BusCreator  Inputs=4  OutDataTypeStr=Bus: vehStatesBus
  Constant{,1..3} (4 alike) : Constant  Value=0
  states : Outport
  wires:
  Constant/1 -> Bus Creator1/2  "Y"
  Constant2/1 -> Bus Creator1/3  "Xdot"
  Constant1/1 -> Bus Creator1/1  "X"
  Bus Creator1/1 -> states/1
  Constant3/1 -> Bus Creator1/4  "u"

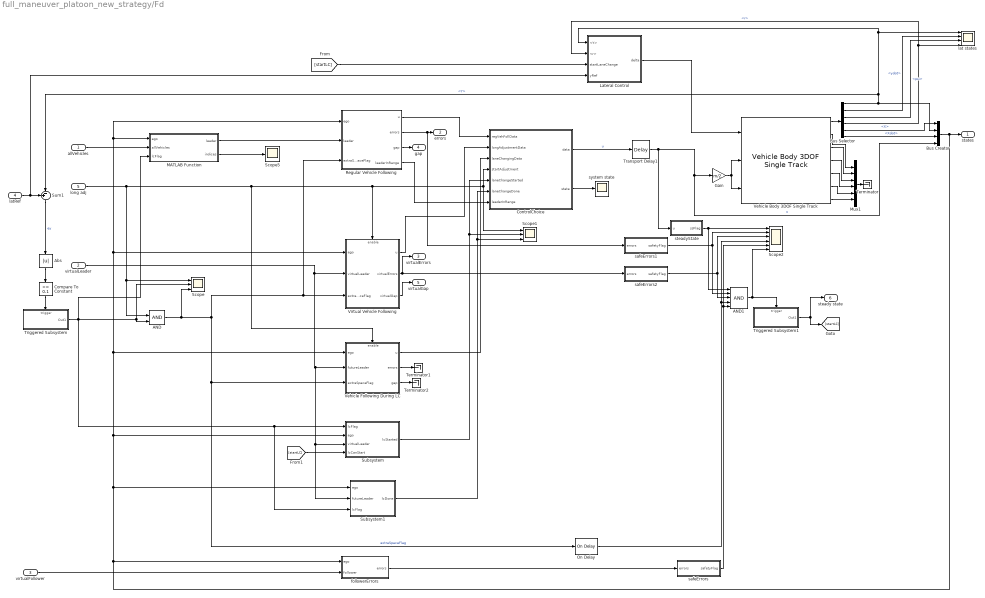
== system full_maneuver_platoon_new_strategy/Fd ==
  allVehicles : Inport
  virtualLeader : Inport  Port=2
  virtualFollower : Inport  Port=3
  latRef : Inport  Port=4
  long adj : Inport  Port=5
  AND : Logic  IconShape=distinctive  AllPortsSameDT=off  OutDataTypeStr=boolean
  AND1 : Logic  Inputs=5  IconShape=distinctive  AllPortsSameDT=off  OutDataTypeStr=boolean
  Abs : Abs
  Bus Creator : BusCreator  Inputs=4  OutDataTypeStr=Bus: vehStatesBus  NonVirtualBus=on
  Bus Selector : BusSelector  OutputSignals=InertFrm.Cg.Disp.Y,BdyFrm.Cg.Vel.ydot,InertFrm.Cg.Ang.psi,BdyFrm.Cg.AngVel.r,InertFrm.RearAxl.Disp.X,InertFrm.RearAxl.Vel.Xdot
  Compare To Constant : simulink/Logic and Bit Operations/Compare To Constant  relop=>=  const=0.1  OutDataTypeStr=boolean
  ControlChoice : Stateflow chart  BlockKeywords=__PRM__SERIALIZED__DATA__:Stateflow Chart,Stateflow Diagram  TreatAsAtomicUnit=on
  Gain : Gain  Gain=m/2
  Lateral Control : Subsystem
  MATLAB Function : MATLAB Function  TreatAsAtomicUnit=on
  Mux1 : Mux  Inputs=6
  On Delay : powerlib_meascontrol/Logic/On Delay  DelayType=On delay  delay=1  ic=0  Ts=0
      settings: SourceProductName=Simscape Electrical
  Regular Vehicle Following : Subsystem
  Scope : Scope  NumInputPorts=3
  Scope1 : Scope  NumInputPorts=3
  Scope2 : Scope  NumInputPorts=6
  Scope5 : Scope
  Subsystem : Subsystem
  Subsystem1 : Subsystem
  Sum1 : Sum  Inputs=+-|
  Terminator : Terminator
  Terminator1 : Terminator
  Terminator2 : Terminator
  Transport Delay1 : TransportDelay  DelayTime=0.01
  Triggered Subsystem : Subsystem  TreatAsAtomicUnit=on
  Triggered Subsystem1 : Subsystem  TreatAsAtomicUnit=on
  Vehicle Body 3DOF Single Track : autolibshared/Vehicle Body 3DOF Single Track  trackMode=Single (bicycle)  inputMode=External longitudinal forces  frontSteerMode=on  rearSteerMode=off  windMode=off  muMode=off  extFMode=off  extMMode=off  extXo=off  extpsio=off  extxdoto=off  extro=off  extYo=off  extTamb=off  extydoto=off  aMode=2  NF=2  NR=2  m=m  a=lf  b=lr  h=0.35  X_o=x0  xdot_o=vx0  CalphaMode=off  sigmaMode=on  d=0  w=[1.4,1.4]  Cy_f=12e3  Cy_r=11e3  sigma_f=.1  sigma_r=.1  alpha_f_brk=[-.1 .1]  Cy_f_data=[-9e3 9e3]  alpha_r_brk=[-.1 .1]  Cy_r_data=[-9e3 9e3]  Y_o=y0  ydot_o=0  Izz=4000  psi_o=0  r_o=0  Af=2  Cd=.3  Cl=.1  Cpm=.1  beta_w=[0:0.01:0.3]  Cs=[0:0.03:0.9]  Cym=[0:0.01:0.3]  Pabs=101325  Tair=273  g=9.81  mu=1  xdot_tol=.01  Fznom=5000  Fxtire_sat=7e4  Fytire_sat=7e4  longOff=0  latOff=0  vertOff=0  wrapAng=off
      settings: SourceProductName=Powertrain Blockset  SourceProductBaseCode=PW
  Vehicle Following During LC : Subsystem  TreatAsAtomicUnit=on
  Virtual Vehicle Following : Subsystem  TreatAsAtomicUnit=on
  followerErrors : Subsystem
  lat states : Scope  NumInputPorts=4
  safeErrors : Subsystem
  safeErrors1 : Subsystem
  safeErrors2 : Subsystem
  steadyState : Subsystem
  system state : Scope
  states : Outport
  errors : Outport  Port=2
  virtualErrors : Outport  Port=3
  gap : Outport  Port=4
  virtualGap : Outport  Port=5
  steady state : Outport  Port=6
  wires:
  Virtual Vehicle Following/2(virtualErrors) -> virtualErrors/1, safeErrors2/1(errors)
  Sum1/1 -> Abs/1  "ey"
  Transport Delay1/1 -> steadyState/1(u), Bus Creator/4, Gain/1  "u"
  virtualLeader/1 -> Subsystem1/2(futureLeader), Subsystem/3(virtualLeader), Vehicle Following During LC/2(futureLeader), Virtual Vehicle Following/2(virtualLeader)
  On Delay/1 -> Scope2/4, AND1/4
  long adj/1 -> Vehicle Following During LC/Enable, Virtual Vehicle Following/Enable, Scope1/1, ControlChoice/4(startAdjustment), Scope/1, AND/1
  AND1/1 -> Triggered Subsystem1/Trigger, Scope2/6
  Bus Creator/1 -> states/1, Subsystem1/1(ego), Regular Vehicle Following/1(ego), MATLAB Function/1(ego), Virtual Vehicle Following/1(ego), Vehicle Following During LC/1(ego), Subsystem/2(ego), followerErrors/1(ego)
  ControlChoice/1(data) -> Transport Delay1/1  "u"
  latRef/1 -> Lateral Control/4(yRef), Sum1/1
  Bus Selector/4 -> Lateral Control/2(<r>), lat states/4  "<r>"
  Bus Selector/3 -> lat states/3  "<psi>"
  Bus Selector/2 -> lat states/2  "<ydot>"
  Bus Selector/1 -> Lateral Control/1(<Y>), lat states/1, Sum1/2, Bus Creator/2  "<Y>"
  Mux1/1 -> Terminator/1
  Vehicle Body 3DOF Single Track/7 -> Mux1/6
  Vehicle Body 3DOF Single Track/6 -> Mux1/5
  Vehicle Body 3DOF Single Track/5 -> Mux1/4
  Vehicle Body 3DOF Single Track/2 -> Mux1/1
  Vehicle Body 3DOF Single Track/3 -> Mux1/2
  Vehicle Body 3DOF Single Track/4 -> Mux1/3
  Vehicle Body 3DOF Single Track/1 -> Bus Selector/1
  Gain/1 -> Vehicle Body 3DOF Single Track/2, Vehicle Body 3DOF Single Track/3
  Bus Selector/5 -> Bus Creator/1  "<X>"
  Bus Selector/6 -> Bus Creator/3  "<Xdot>"
  AND/1 -> Scope/3, Regular Vehicle Following/3(extraSpaceFlag), Virtual Vehicle Following/3(extraSpaceFlag), On Delay/1, Vehicle Following During LC/3(extraSpaceFlag)  "extraSpaceFlag"
  Abs/1 -> Compare To Constant/1
  Compare To Constant/1 -> Triggered Subsystem/Trigger
  allVehicles/1 -> MATLAB Function/2(allVehicles)
  MATLAB Function/1(leader) -> Regular Vehicle Following/2(leader)
  safeErrors/1(safetyFlag) -> Scope2/5, AND1/5
  followerErrors/1(errors) -> safeErrors/1(errors)
  safeErrors1/1(safetyFlag) -> AND1/2, Scope2/2
  safeErrors2/1(safetyFlag) -> Scope2/3, AND1/3
  steadyState/1(ssFlag) -> AND1/1, Scope2/1
  virtualFollower/1 -> followerErrors/2(follower)
  MATLAB Function/2(indices) -> Scope5/1
  Regular Vehicle Following/3(gap) -> gap/1
  Regular Vehicle Following/1(u) -> ControlChoice/1(regVehFollData)
  Virtual Vehicle Following/1(u) -> ControlChoice/2(longAdjustmentData)
  Regular Vehicle Following/2(errors) -> safeErrors1/1(errors), errors/1
  [startLC] -> Lateral Control/3(startLaneChange)
  Lateral Control/1(delta) -> Vehicle Body 3DOF Single Track/1
  Subsystem/1(lcStarted) -> Scope1/2, ControlChoice/5(laneChangeStarted)
  ControlChoice/2(state) -> system state/1
  Vehicle Following During LC/1(u) -> ControlChoice/3(laneChangingData)
  Subsystem1/1(lcDone) -> Scope1/3, ControlChoice/6(laneChangeDone)
  Vehicle Following During LC/2(errors) -> Terminator1/1
  Vehicle Following During LC/3(gap) -> Terminator2/1
  Virtual Vehicle Following/3(virtualGap) -> virtualGap/1
  [startLC] -> Subsystem/4(lcCanStart)
  Triggered Subsystem/1(Out1) -> MATLAB Function/3(lcFlag), Subsystem1/3(lcFlag), Subsystem/1(lcFlag), AND/2, Scope/2
  Triggered Subsystem1/1(Out1) -> steady state/1, [startLC]
  Regular Vehicle Following/4(leaderInRange) -> ControlChoice/7(leaderInRange)
